simulink model "prblm5"  (R2020b)
settings: Solver=VariableStepAuto  StartTime=0.0  StopTime=10.0  RelTol=1e-3
settings Model: Creator=shridhar  LastModifiedBy=shridhar

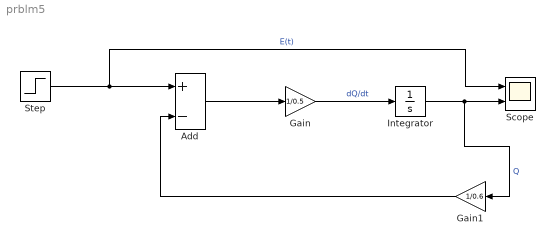
== system prblm5 ==
  Add : Sum  Inputs=+-
  Gain : Gain  Gain=1/0.5
  Gain1 : Gain  Gain=1/0.6
  Integrator : Integrator  InitialCondition=5
  Scope : Scope  NumInputPorts=2
  Step : Step  Time=5  SampleTime=0
  wires:
  Gain1/1 -> Add/2
  Integrator/1 -> Gain1/1, Scope/2  "Q"
  Add/1 -> Gain/1
  Step/1 -> Scope/1, Add/1  "E(t)"
  Gain/1 -> Integrator/1  "dQ/dt"
